simulink model "Pendel"  (R2013a)
settings: Solver=ode3  StartTime=0.0  StopTime=20  FixedStep=0.00001  RelTol=1e-3
undefined symbols (not defined in the file or in its folder): d, g, l, m
settings Model: Creator=Jan  LastModifiedBy=Jan

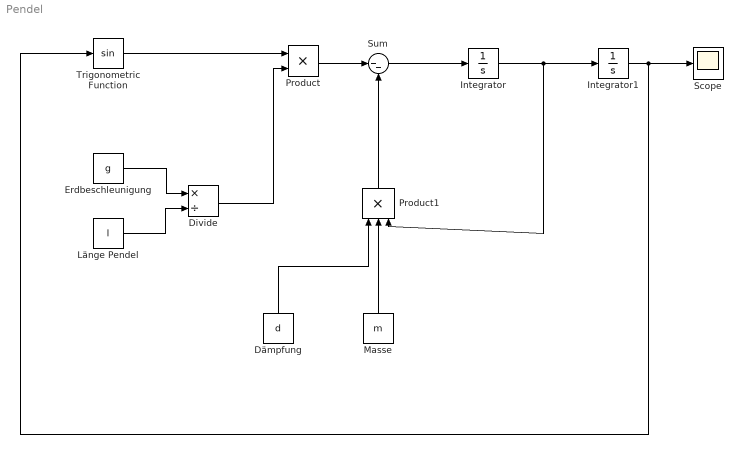
== system Pendel ==
  Divide : Product  Inputs=*/
  Dämpfung : Constant  Value=d
  Erdbeschleunigung : Constant  Value=g
  Integrator : Integrator
  Integrator1 : Integrator  InitialCondition=(40*pi)/180
  Länge Pendel : Constant  Value=l
  Masse : Constant  Value=m
  Product : Product
  Product1 : Product  Inputs=3
  Scope : Scope
  Sum : Sum  Inputs=|--
  Trigonometric Function : Trigonometry
  wires:
  Trigonometric Function/1 -> Product/1
  Divide/1 -> Product/2
  Erdbeschleunigung/1 -> Divide/1
  Länge Pendel/1 -> Divide/2
  Product/1 -> Sum/1
  Product1/1 -> Sum/2
  Masse/1 -> Product1/2
  Dämpfung/1 -> Product1/1
  Sum/1 -> Integrator/1
  Integrator/1 -> Integrator1/1, Product1/3
  Integrator1/1 -> Scope/1, Trigonometric Function/1
